simulink model "freqDectect"  (R2018b)
settings: Solver=VariableStepAuto  StartTime=0.0  StopTime=inf  RelTol=1e-3
libraries: dspfdesign x2, audiosources x1, dspxfrm3 x1, dspsigops x1
settings Model: Creator=emilyearl  LastModifiedBy=emilyearl

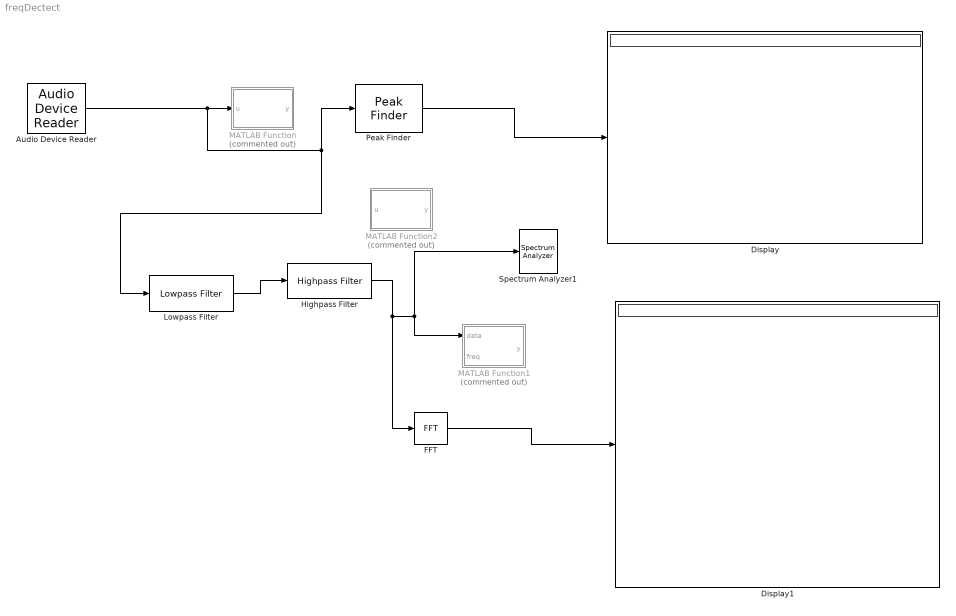
== system freqDectect ==
  Audio Device Reader : audiosources/Audio Device Reader  Driver=CoreAudio  Device=Built-in Microphone  SampleRate=44100  NumChannels=1  SamplesPerFrame=100  BitDepth=16-bit integer  NumBuffers=10  DefaultInputChannelMapping=on  InputChannelMapping=1:2  OutputNumOverrunSamples=off  OutputDataType=double  DriverIdx=5  DeviceWarnFlag=''
      settings: SourceProductName=Audio System Toolbox  SourceProductBaseCode=AU
  Display : Display
  Display1 : Display
  FFT : dspxfrm3/FFT  FFTImplementation=Auto  CompMethod=Table lookup  TableOpt=NEW  TableOptActive=Speed  BitRevOrder=off  Normalize=off  InheritFFTLength=on  FFTLength=64  WrapInput=on  roundingMode=Floor  overflowMode=off  firstCoeffDataTypeStr=Inherit: Same word length as input  firstCoeffLastDataTypeStr=Inherit: Same word length as input  outputMin=[]  outputMax=[]
  Highpass Filter : dspfdesign/Highpass Filter  FilterType=FIR  DesignForMinimumOrder=on  FilterOrder=50  StopbandFrequency=100  PassbandFrequency=200  StopbandAttenuation=80  PassbandRipple=0.1  InheritSampleRate=off  SampleRate=44100  SimulateUsing=Interpreted execution  roundingMode=Floor  coeffsDataTypeStr=fixdt(1,16)
      settings: SourceProductName=DSP System Toolbox
  Lowpass Filter : dspfdesign/Lowpass Filter  FilterType=FIR  DesignForMinimumOrder=on  FilterOrder=50  PassbandFrequency=6e3  StopbandFrequency=7e3  PassbandRipple=0.1  StopbandAttenuation=80  InheritSampleRate=off  SampleRate=44100  SimulateUsing=Interpreted execution  roundingMode=Floor  coeffsDataTypeStr=fixdt(1,16)
  MATLAB Function : MATLAB Function  Commented=on  TreatAsAtomicUnit=on
  MATLAB Function1 : MATLAB Function  Commented=on  TreatAsAtomicUnit=on
  MATLAB Function2 : MATLAB Function  Commented=on  TreatAsAtomicUnit=on
  Peak Finder : dspsigops/Peak Finder  polarity=Maxima  outputIdx=on  outputVal=on  maxPeaks=40  NoiseDistinguish=on  thresh=0  roundingMode=Floor  overflowMode=off
      settings: SourceProductName=DSP System Toolbox  SourceProductBaseCode=DS  allowOverrides=off
  Spectrum Analyzer1 : SpectrumAnalyzer
  wires:
  Audio Device Reader/1 -> Peak Finder/1, Lowpass Filter/1, MATLAB Function/1(u)
  Peak Finder/2 -> Display/1
  Lowpass Filter/1 -> Highpass Filter/1
  Highpass Filter/1 -> FFT/1, Spectrum Analyzer1/1, MATLAB Function1/1(data)
  FFT/1 -> Display1/1

== matlab function freqDectect/MATLAB Function1 ==
  data: data input; y output; freq input
function y = fcn(data, freq)

[pks,frqs] = findpeaks(data,freq);
y = 0
for i = 1:length(data)
    if (data(i) == yval)
       y = i
    end
end

== matlab function freqDectect/MATLAB Function ==
  data: u input; y output
function y = fcn(u)
recorder = audiorecorder;
rec = getaudiodata(recorder);
display()

== matlab function freqDectect/MATLAB Function2 ==
  data: u input; y output
function y = fcn(u)
span
y = u;
